simulink model "dota2_CGT"  (R2021a)
settings: Solver=VariableStepAuto  StartTime=0.0  StopTime=10.0  RelTol=1e-3
libraries: pid_lib x5, simulink x1
settings Model: Creator=srika  LastModifiedBy=srika
settings HardwareCC: TargetBitPerPointer=64  TargetBitPerSizeT=64  TargetBitPerPtrDiffT=64  TargetLongLongMode=on  TargetIntDivRoundTo=Zero  TargetEndianess=LittleEndian  TargetWordSize=64  TargetHWDeviceType=MATLAB Host  ProdEqTarget=off
settings SFSimCC: SimParseCustomCode=off
settings RTWCC: Description=Rapid Simulation Target  SystemTargetFile=rsim.tlc  TemplateMakefile=rsim_default_tmf
settings RSimTargetCC: TargetLangStandard=C99 (ISO)

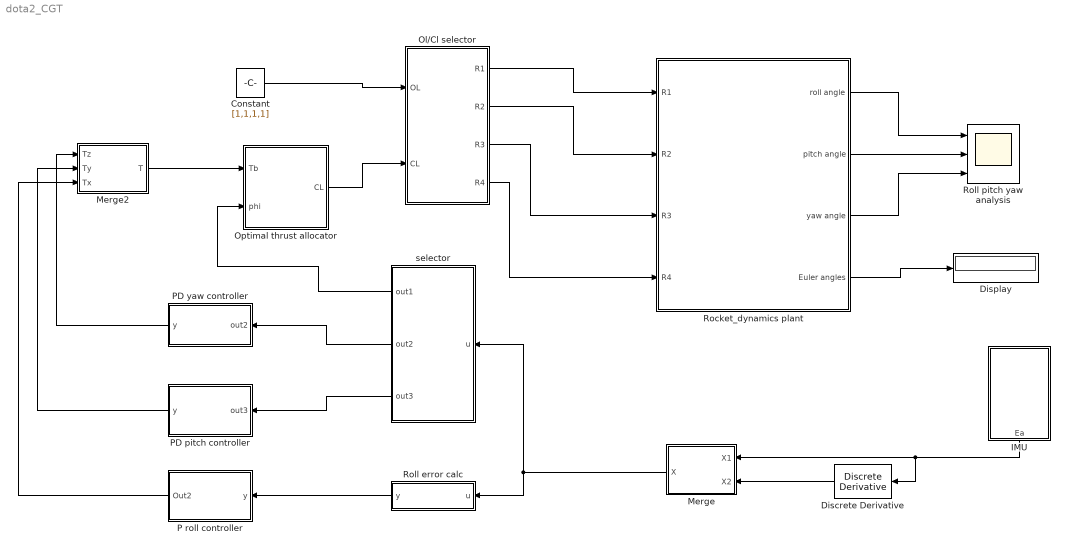
== system dota2_CGT ==
  " P roll controller" : Subsystem
  Constant : Constant  Value=[1,1,1,1]  VectorParams1D=off
  Discrete Derivative : simulink/Discrete/Discrete Derivative  gainval=1.0  ICPrevScaledInput=0.0  OutMin=[]  OutMax=[]  OutDataType=fixdt(1, 16)  OutScaling=2^-10  DoSatur=off
  Display : Display
  "IMU " : MATLAB Function  TreatAsAtomicUnit=on
  Merge : MATLAB Function  TreatAsAtomicUnit=on
  Merge2 : MATLAB Function  TreatAsAtomicUnit=on
  "Ol/Cl selector " : MATLAB Function  TreatAsAtomicUnit=on
  Optimal thrust allocator : Subsystem
  PD pitch controller : Subsystem
  PD yaw controller : Subsystem
  Rocket_dynamics plant : Subsystem
  Roll error calc : MATLAB Function  TreatAsAtomicUnit=on
  Roll pitch yaw analysis : Scope  NumInputPorts=3
  "selector " : MATLAB Function  TreatAsAtomicUnit=on
  wires:
  "IMU "/1(Ea) -> Merge/1(X1), Discrete Derivative/1
  Roll error calc/1(y) -> " P roll controller"/1(y)
  "selector "/1(out1) -> Optimal thrust allocator/2(phi)
  "selector "/2(out2) -> PD yaw controller/1(out2)
  "selector "/3(out3) -> PD pitch controller/1(out3)
  PD yaw controller/1(y) -> Merge2/1(Tz)
  PD pitch controller/1(y) -> Merge2/2(Ty)
  " P roll controller"/1(Out2) -> Merge2/3(Tx)
  Optimal thrust allocator/1(CL) -> "Ol/Cl selector "/2(CL)
  Constant/1 -> "Ol/Cl selector "/1(OL)
  "Ol/Cl selector "/1(R1) -> Rocket_dynamics plant/1(R1)
  "Ol/Cl selector "/2(R2) -> Rocket_dynamics plant/2(R2)
  "Ol/Cl selector "/3(R3) -> Rocket_dynamics plant/3(R3)
  "Ol/Cl selector "/4(R4) -> Rocket_dynamics plant/4(R4)
  Rocket_dynamics plant/1(roll angle) -> Roll pitch yaw analysis/1
  Rocket_dynamics plant/2(pitch angle) -> Roll pitch yaw analysis/2
  Rocket_dynamics plant/3(yaw angle) -> Roll pitch yaw analysis/3
  Merge2/1(T) -> Optimal thrust allocator/1(Tb)
  Discrete Derivative/1 -> Merge/2(X2)
  Merge/1(X) -> "selector "/1(u), Roll error calc/1(u)
  Rocket_dynamics plant/4(Euler angles) -> Display/1

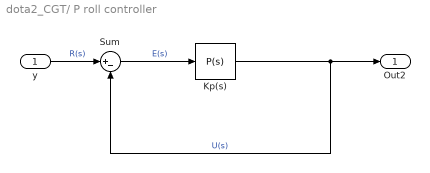
== system dota2_CGT/ P roll controller ==
  y : Inport
  Kp(s) : pid_lib/PID Controller  Controller=P  Form=Parallel  TimeDomain=Continuous-time  UseExternalTs=off  SampleTime=-1  IntegratorMethod=Forward Euler  FilterMethod=Forward Euler  ControllerParametersSource=internal  P=0.002063  I=1  D=5  UseFilter=on  N=100  TunerSelectOption=Transfer Function Based (PID Tuner App)  InitialConditionSource=internal  InitialConditionForIntegrator=0  InitialConditionForFilter=0  DifferentiatorICPrevScaledInput=0  ExternalReset=none  TrackingMode=off  Kt=1  LimitOutput=off  SatLimitsSource=internal  UpperSaturationLimit=inf  LowerSaturationLimit=-inf  LinearizeAsGain=on  AntiWindupMode=none  Kb=1  POutMin=[]  POutMax=[]  IOutMin=[]  IOutMax=[]  DOutMin=[]  DOutMax=[]  NOutMin=[]  NOutMax=[]  SumOutMin=[]  SumOutMax=[]  SaturationOutMin=[]  SaturationOutMax=[]  PParamMin=[]  PParamMax=[]  IParamMin=[]  IParamMax=[]  DParamMin=[]  DParamMax=[]  NParamMin=[]  NParamMax=[]  KbParamMin=[]  KbParamMax=[]  KtParamMin=[]  KtParamMax=[]  KbOutMin=[]  KbOutMax=[]  KtOutMin=[]  KtOutMax=[]  IntegratorOutMin=[]  IntegratorOutMax=[]  FilterOutMin=[]  FilterOutMax=[]  SumI1OutMin=[]  SumI1OutMax=[]  SumI2OutMin=[]  SumI2OutMax=[]  SumI3OutMin=[]  SumI3OutMax=[]  SumI4OutMin=[]  SumI4OutMax=[]  SumDOutMin=[]  SumDOutMax=[]  DifferentiatorOutMin=[]  DifferentiatorOutMax=[]  FilterDiffOutCoefMin=[]  FilterDiffOutCoefMax=[]  ReciprocalOutMin=[]  ReciprocalOutMax=[]  SumDenOutMin=[]  SumDenOutMax=[]  SumNumOutMin=[]  SumNumOutMax=[]  DivideOutMin=[]  DivideOutMax=[]  UdiffTsProdOutMin=[]  UdiffTsProdOutMax=[]  NTsProdOutMin=[]  NTsProdOutMax=[]  UintegralTsProdOutMin=[]  UintegralTsProdOutMax=[]  UngainTsProdOutMin=[]  UngainTsProdOutMax=[]  IntegratorContinuousStateAttributes=''  IntegratorStateMustResolveToSignalObject=off  IntegratorRTWStateStorageClass=Auto  FilterContinuousStateAttributes=''  FilterStateMustResolveToSignalObject=off  FilterRTWStateStorageClass=Auto  ParallelPVariant=InternalParameters  IdealPVariant=Disabled  IVariant=Disabled  DVariant=Disabled  IntegratorVariant=Disabled  SatVariant=Disabled  AWVariant=Disabled  PCopyVariant=Disabled  TRVariant=Disabled  FdbkBlocksVariant=Forward  IdealPFdbkVariant=Disabled  SatFdbkVariant=Disabled  DerivativeFilterVariant=Disabled  NVariant=Disabled  NCopyVariant=Disabled_SignalSpec  FilterICVariant=Disabled  IntegratorICVariant=Disabled  ExternalResetVariant=Disabled  TRSumVariant=Passthrough  SumFdbkVariant=Disabled  SumVariant=Passthrough_P  TsampFilterVariant=InternalTs  TsampNgainVariant=Passthrough  TsampIntegralVariant=Disabled_SignalSpec  ExternalSaturationOutDataTypeStr=Inherit: Same as second input
  Sum : Sum  Inputs=|+-
  Out2 : Outport
  wires:
  Sum/1 -> Kp(s)/1  "E(s)"
  Kp(s)/1 -> Sum/2, Out2/1  "U(s)"
  y/1 -> Sum/1  "R(s)"

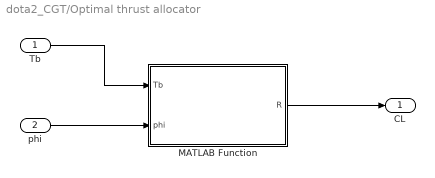
== system dota2_CGT/Optimal thrust allocator ==
  Tb : Inport
  phi : Inport  Port=2
  MATLAB Function : MATLAB Function  TreatAsAtomicUnit=on
  CL : Outport
  wires:
  Tb/1 -> MATLAB Function/1(Tb)
  phi/1 -> MATLAB Function/2(phi)
  MATLAB Function/1(R) -> CL/1

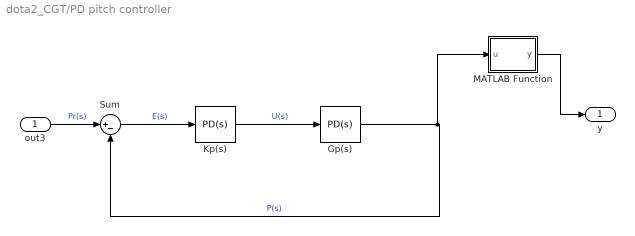
== system dota2_CGT/PD pitch controller ==
  out3 : Inport
  Gp(s) : pid_lib/PID Controller  Controller=PD  Form=Parallel  TimeDomain=Continuous-time  UseExternalTs=off  SampleTime=-1  IntegratorMethod=Forward Euler  FilterMethod=Forward Euler  ControllerParametersSource=internal  P=3  I=1  D=15  UseFilter=on  N=100  TunerSelectOption=Transfer Function Based (PID Tuner App)  InitialConditionSource=internal  InitialConditionForIntegrator=0  InitialConditionForFilter=0  DifferentiatorICPrevScaledInput=0  ExternalReset=none  TrackingMode=off  Kt=1  LimitOutput=off  SatLimitsSource=internal  UpperSaturationLimit=inf  LowerSaturationLimit=-inf  LinearizeAsGain=on  AntiWindupMode=none  Kb=1  POutMin=[]  POutMax=[]  IOutMin=[]  IOutMax=[]  DOutMin=[]  DOutMax=[]  NOutMin=[]  NOutMax=[]  SumOutMin=[]  SumOutMax=[]  SaturationOutMin=[]  SaturationOutMax=[]  PParamMin=[]  PParamMax=[]  IParamMin=[]  IParamMax=[]  DParamMin=[]  DParamMax=[]  NParamMin=[]  NParamMax=[]  KbParamMin=[]  KbParamMax=[]  KtParamMin=[]  KtParamMax=[]  KbOutMin=[]  KbOutMax=[]  KtOutMin=[]  KtOutMax=[]  IntegratorOutMin=[]  IntegratorOutMax=[]  FilterOutMin=[]  FilterOutMax=[]  SumI1OutMin=[]  SumI1OutMax=[]  SumI2OutMin=[]  SumI2OutMax=[]  SumI3OutMin=[]  SumI3OutMax=[]  SumI4OutMin=[]  SumI4OutMax=[]  SumDOutMin=[]  SumDOutMax=[]  DifferentiatorOutMin=[]  DifferentiatorOutMax=[]  FilterDiffOutCoefMin=[]  FilterDiffOutCoefMax=[]  ReciprocalOutMin=[]  ReciprocalOutMax=[]  SumDenOutMin=[]  SumDenOutMax=[]  SumNumOutMin=[]  SumNumOutMax=[]  DivideOutMin=[]  DivideOutMax=[]  UdiffTsProdOutMin=[]  UdiffTsProdOutMax=[]  NTsProdOutMin=[]  NTsProdOutMax=[]  UintegralTsProdOutMin=[]  UintegralTsProdOutMax=[]  UngainTsProdOutMin=[]  UngainTsProdOutMax=[]  IntegratorContinuousStateAttributes=''  IntegratorStateMustResolveToSignalObject=off  IntegratorRTWStateStorageClass=Auto  FilterContinuousStateAttributes=''  FilterStateMustResolveToSignalObject=off  FilterRTWStateStorageClass=Auto  ParallelPVariant=InternalParameters  IdealPVariant=Disabled  IVariant=Disabled  DVariant=InternalParameters  IntegratorVariant=Disabled  SatVariant=Disabled  AWVariant=Disabled  PCopyVariant=Disabled  TRVariant=Disabled  FdbkBlocksVariant=Forward  IdealPFdbkVariant=Disabled  SatFdbkVariant=Disabled  DerivativeFilterVariant=ContFilter  NVariant=InternalParameters  NCopyVariant=Disabled  FilterICVariant=InternalICsFilter  IntegratorICVariant=Disabled  ExternalResetVariant=Disabled  TRSumVariant=Passthrough  SumFdbkVariant=Disabled  SumVariant=Sum_PD  TsampFilterVariant=InternalTs  TsampNgainVariant=Passthrough  TsampIntegralVariant=Disabled_SignalSpec  ExternalSaturationOutDataTypeStr=Inherit: Same as second input
  Kp(s) : pid_lib/PID Controller  Controller=PD  Form=Parallel  TimeDomain=Continuous-time  UseExternalTs=off  SampleTime=-1  IntegratorMethod=Forward Euler  FilterMethod=Forward Euler  ControllerParametersSource=internal  P=3  I=1  D=5  UseFilter=on  N=100  TunerSelectOption=Transfer Function Based (PID Tuner App)  InitialConditionSource=internal  InitialConditionForIntegrator=0  InitialConditionForFilter=0  DifferentiatorICPrevScaledInput=0  ExternalReset=none  TrackingMode=off  Kt=1  LimitOutput=off  SatLimitsSource=internal  UpperSaturationLimit=inf  LowerSaturationLimit=-inf  LinearizeAsGain=on  AntiWindupMode=none  Kb=1  POutMin=[]  POutMax=[]  IOutMin=[]  IOutMax=[]  DOutMin=[]  DOutMax=[]  NOutMin=[]  NOutMax=[]  SumOutMin=[]  SumOutMax=[]  SaturationOutMin=[]  SaturationOutMax=[]  PParamMin=[]  PParamMax=[]  IParamMin=[]  IParamMax=[]  DParamMin=[]  DParamMax=[]  NParamMin=[]  NParamMax=[]  KbParamMin=[]  KbParamMax=[]  KtParamMin=[]  KtParamMax=[]  KbOutMin=[]  KbOutMax=[]  KtOutMin=[]  KtOutMax=[]  IntegratorOutMin=[]  IntegratorOutMax=[]  FilterOutMin=[]  FilterOutMax=[]  SumI1OutMin=[]  SumI1OutMax=[]  SumI2OutMin=[]  SumI2OutMax=[]  SumI3OutMin=[]  SumI3OutMax=[]  SumI4OutMin=[]  SumI4OutMax=[]  SumDOutMin=[]  SumDOutMax=[]  DifferentiatorOutMin=[]  DifferentiatorOutMax=[]  FilterDiffOutCoefMin=[]  FilterDiffOutCoefMax=[]  ReciprocalOutMin=[]  ReciprocalOutMax=[]  SumDenOutMin=[]  SumDenOutMax=[]  SumNumOutMin=[]  SumNumOutMax=[]  DivideOutMin=[]  DivideOutMax=[]  UdiffTsProdOutMin=[]  UdiffTsProdOutMax=[]  NTsProdOutMin=[]  NTsProdOutMax=[]  UintegralTsProdOutMin=[]  UintegralTsProdOutMax=[]  UngainTsProdOutMin=[]  UngainTsProdOutMax=[]  IntegratorContinuousStateAttributes=''  IntegratorStateMustResolveToSignalObject=off  IntegratorRTWStateStorageClass=Auto  FilterContinuousStateAttributes=''  FilterStateMustResolveToSignalObject=off  FilterRTWStateStorageClass=Auto  ParallelPVariant=InternalParameters  IdealPVariant=Disabled  IVariant=Disabled  DVariant=InternalParameters  IntegratorVariant=Disabled  SatVariant=Disabled  AWVariant=Disabled  PCopyVariant=Disabled  TRVariant=Disabled  FdbkBlocksVariant=Forward  IdealPFdbkVariant=Disabled  SatFdbkVariant=Disabled  DerivativeFilterVariant=ContFilter  NVariant=InternalParameters  NCopyVariant=Disabled  FilterICVariant=InternalICsFilter  IntegratorICVariant=Disabled  ExternalResetVariant=Disabled  TRSumVariant=Passthrough  SumFdbkVariant=Disabled  SumVariant=Sum_PD  TsampFilterVariant=InternalTs  TsampNgainVariant=Passthrough  TsampIntegralVariant=Disabled_SignalSpec  ExternalSaturationOutDataTypeStr=Inherit: Same as second input
  MATLAB Function : MATLAB Function  TreatAsAtomicUnit=on
  Sum : Sum  Inputs=|+-
  y : Outport
  wires:
  Gp(s)/1 -> MATLAB Function/1(u), Sum/2  "P(s)"
  Sum/1 -> Kp(s)/1  "E(s)"
  Kp(s)/1 -> Gp(s)/1  "U(s)"
  out3/1 -> Sum/1  "Pr(s)"
  MATLAB Function/1(y) -> y/1

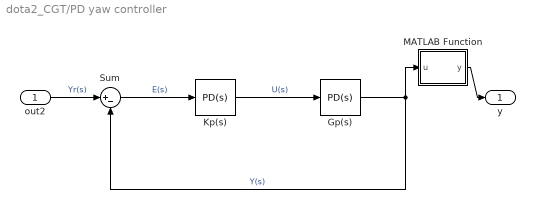
== system dota2_CGT/PD yaw controller ==
  out2 : Inport
  Gp(s) : pid_lib/PID Controller  Controller=PD  Form=Parallel  TimeDomain=Continuous-time  UseExternalTs=off  SampleTime=-1  IntegratorMethod=Forward Euler  FilterMethod=Forward Euler  ControllerParametersSource=internal  P=3  I=1  D=15  UseFilter=on  N=100  TunerSelectOption=Transfer Function Based (PID Tuner App)  InitialConditionSource=internal  InitialConditionForIntegrator=0  InitialConditionForFilter=0  DifferentiatorICPrevScaledInput=0  ExternalReset=none  TrackingMode=off  Kt=1  LimitOutput=off  SatLimitsSource=internal  UpperSaturationLimit=inf  LowerSaturationLimit=-inf  LinearizeAsGain=on  AntiWindupMode=none  Kb=1  POutMin=[]  POutMax=[]  IOutMin=[]  IOutMax=[]  DOutMin=[]  DOutMax=[]  NOutMin=[]  NOutMax=[]  SumOutMin=[]  SumOutMax=[]  SaturationOutMin=[]  SaturationOutMax=[]  PParamMin=[]  PParamMax=[]  IParamMin=[]  IParamMax=[]  DParamMin=[]  DParamMax=[]  NParamMin=[]  NParamMax=[]  KbParamMin=[]  KbParamMax=[]  KtParamMin=[]  KtParamMax=[]  KbOutMin=[]  KbOutMax=[]  KtOutMin=[]  KtOutMax=[]  IntegratorOutMin=[]  IntegratorOutMax=[]  FilterOutMin=[]  FilterOutMax=[]  SumI1OutMin=[]  SumI1OutMax=[]  SumI2OutMin=[]  SumI2OutMax=[]  SumI3OutMin=[]  SumI3OutMax=[]  SumI4OutMin=[]  SumI4OutMax=[]  SumDOutMin=[]  SumDOutMax=[]  DifferentiatorOutMin=[]  DifferentiatorOutMax=[]  FilterDiffOutCoefMin=[]  FilterDiffOutCoefMax=[]  ReciprocalOutMin=[]  ReciprocalOutMax=[]  SumDenOutMin=[]  SumDenOutMax=[]  SumNumOutMin=[]  SumNumOutMax=[]  DivideOutMin=[]  DivideOutMax=[]  UdiffTsProdOutMin=[]  UdiffTsProdOutMax=[]  NTsProdOutMin=[]  NTsProdOutMax=[]  UintegralTsProdOutMin=[]  UintegralTsProdOutMax=[]  UngainTsProdOutMin=[]  UngainTsProdOutMax=[]  IntegratorContinuousStateAttributes=''  IntegratorStateMustResolveToSignalObject=off  IntegratorRTWStateStorageClass=Auto  FilterContinuousStateAttributes=''  FilterStateMustResolveToSignalObject=off  FilterRTWStateStorageClass=Auto  ParallelPVariant=InternalParameters  IdealPVariant=Disabled  IVariant=Disabled  DVariant=InternalParameters  IntegratorVariant=Disabled  SatVariant=Disabled  AWVariant=Disabled  PCopyVariant=Disabled  TRVariant=Disabled  FdbkBlocksVariant=Forward  IdealPFdbkVariant=Disabled  SatFdbkVariant=Disabled  DerivativeFilterVariant=ContFilter  NVariant=InternalParameters  NCopyVariant=Disabled  FilterICVariant=InternalICsFilter  IntegratorICVariant=Disabled  ExternalResetVariant=Disabled  TRSumVariant=Passthrough  SumFdbkVariant=Disabled  SumVariant=Sum_PD  TsampFilterVariant=InternalTs  TsampNgainVariant=Passthrough  TsampIntegralVariant=Disabled_SignalSpec  ExternalSaturationOutDataTypeStr=Inherit: Same as second input
  Kp(s) : pid_lib/PID Controller  Controller=PD  Form=Parallel  TimeDomain=Continuous-time  UseExternalTs=off  SampleTime=-1  IntegratorMethod=Forward Euler  FilterMethod=Forward Euler  ControllerParametersSource=internal  P=3  I=1  D=5  UseFilter=on  N=100  TunerSelectOption=Transfer Function Based (PID Tuner App)  InitialConditionSource=internal  InitialConditionForIntegrator=0  InitialConditionForFilter=0  DifferentiatorICPrevScaledInput=0  ExternalReset=none  TrackingMode=off  Kt=1  LimitOutput=off  SatLimitsSource=internal  UpperSaturationLimit=inf  LowerSaturationLimit=-inf  LinearizeAsGain=on  AntiWindupMode=none  Kb=1  POutMin=[]  POutMax=[]  IOutMin=[]  IOutMax=[]  DOutMin=[]  DOutMax=[]  NOutMin=[]  NOutMax=[]  SumOutMin=[]  SumOutMax=[]  SaturationOutMin=[]  SaturationOutMax=[]  PParamMin=[]  PParamMax=[]  IParamMin=[]  IParamMax=[]  DParamMin=[]  DParamMax=[]  NParamMin=[]  NParamMax=[]  KbParamMin=[]  KbParamMax=[]  KtParamMin=[]  KtParamMax=[]  KbOutMin=[]  KbOutMax=[]  KtOutMin=[]  KtOutMax=[]  IntegratorOutMin=[]  IntegratorOutMax=[]  FilterOutMin=[]  FilterOutMax=[]  SumI1OutMin=[]  SumI1OutMax=[]  SumI2OutMin=[]  SumI2OutMax=[]  SumI3OutMin=[]  SumI3OutMax=[]  SumI4OutMin=[]  SumI4OutMax=[]  SumDOutMin=[]  SumDOutMax=[]  DifferentiatorOutMin=[]  DifferentiatorOutMax=[]  FilterDiffOutCoefMin=[]  FilterDiffOutCoefMax=[]  ReciprocalOutMin=[]  ReciprocalOutMax=[]  SumDenOutMin=[]  SumDenOutMax=[]  SumNumOutMin=[]  SumNumOutMax=[]  DivideOutMin=[]  DivideOutMax=[]  UdiffTsProdOutMin=[]  UdiffTsProdOutMax=[]  NTsProdOutMin=[]  NTsProdOutMax=[]  UintegralTsProdOutMin=[]  UintegralTsProdOutMax=[]  UngainTsProdOutMin=[]  UngainTsProdOutMax=[]  IntegratorContinuousStateAttributes=''  IntegratorStateMustResolveToSignalObject=off  IntegratorRTWStateStorageClass=Auto  FilterContinuousStateAttributes=''  FilterStateMustResolveToSignalObject=off  FilterRTWStateStorageClass=Auto  ParallelPVariant=InternalParameters  IdealPVariant=Disabled  IVariant=Disabled  DVariant=InternalParameters  IntegratorVariant=Disabled  SatVariant=Disabled  AWVariant=Disabled  PCopyVariant=Disabled  TRVariant=Disabled  FdbkBlocksVariant=Forward  IdealPFdbkVariant=Disabled  SatFdbkVariant=Disabled  DerivativeFilterVariant=ContFilter  NVariant=InternalParameters  NCopyVariant=Disabled  FilterICVariant=InternalICsFilter  IntegratorICVariant=Disabled  ExternalResetVariant=Disabled  TRSumVariant=Passthrough  SumFdbkVariant=Disabled  SumVariant=Sum_PD  TsampFilterVariant=InternalTs  TsampNgainVariant=Passthrough  TsampIntegralVariant=Disabled_SignalSpec  ExternalSaturationOutDataTypeStr=Inherit: Same as second input
  MATLAB Function : MATLAB Function  TreatAsAtomicUnit=on
  Sum : Sum  Inputs=|+-
  y : Outport
  wires:
  Kp(s)/1 -> Gp(s)/1  "U(s)"
  Sum/1 -> Kp(s)/1  "E(s)"
  out2/1 -> Sum/1  "Yr(s)"
  Gp(s)/1 -> MATLAB Function/1(u), Sum/2  "Y(s)"
  MATLAB Function/1(y) -> y/1

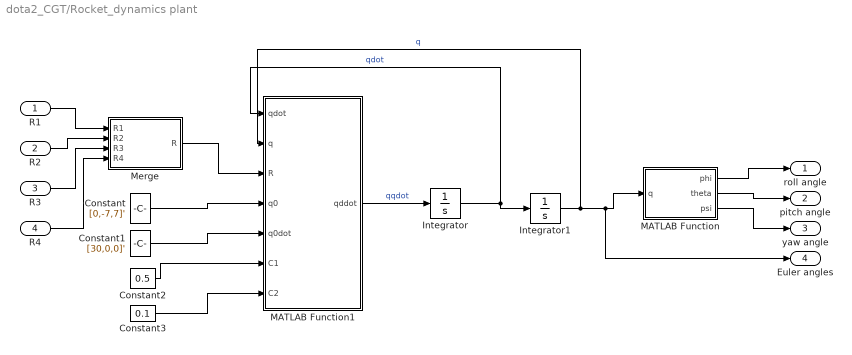
== system dota2_CGT/Rocket_dynamics plant ==
  R1 : Inport
  R2 : Inport  Port=2
  R3 : Inport  Port=3
  R4 : Inport  Port=4
  Constant : Constant  Value=[0,-7,7]'
  Constant1 : Constant  Value=[30,0,0]'
  Constant2 : Constant  Value=0.5
  Constant3 : Constant  Value=0.1
  Integrator : Integrator
  Integrator1 : Integrator
  MATLAB Function : MATLAB Function  TreatAsAtomicUnit=on
  MATLAB Function1 : MATLAB Function  TreatAsAtomicUnit=on
  Merge : MATLAB Function  TreatAsAtomicUnit=on
  roll angle : Outport
  pitch angle : Outport  Port=2
  yaw angle : Outport  Port=3
  Euler angles : Outport  Port=4
  wires:
  Constant3/1 -> MATLAB Function1/7(C2)
  Constant1/1 -> MATLAB Function1/5(q0dot)
  Merge/1(R) -> MATLAB Function1/3(R)
  Integrator/1 -> Integrator1/1, MATLAB Function1/1(qdot)  "qdot"
  R2/1 -> Merge/2(R2)
  MATLAB Function/2(theta) -> pitch angle/1
  Integrator1/1 -> MATLAB Function1/2(q), Euler angles/1, MATLAB Function/1(q)  "q"
  MATLAB Function/1(phi) -> roll angle/1
  MATLAB Function/3(psi) -> yaw angle/1
  R1/1 -> Merge/1(R1)
  R3/1 -> Merge/3(R3)
  MATLAB Function1/1(qddot) -> Integrator/1  "qqdot"
  Constant2/1 -> MATLAB Function1/6(C1)
  Constant/1 -> MATLAB Function1/4(q0)
  R4/1 -> Merge/4(R4)

== matlab function dota2_CGT/PD yaw controller/MATLAB Function ==
  data: u input; y output
function y = fcn(u)

y = u(1);

== matlab function dota2_CGT/PD pitch controller/MATLAB Function ==
  data: u input; y output
function y = fcn(u)

y = u(1);

== matlab function dota2_CGT/IMU  ==
  data: Ea output
function Ea= imu()
    %data_log=zeros(1,20);
    %data_log = readtable("imu_data.csv");
    %Ea=data_log(1,3:5);
    Ea=[3.14/6,3.14/4,3.14/8];

== matlab function dota2_CGT/Optimal thrust allocator/MATLAB Function ==
  data: Tb input; R output; phi input
function R = fcn(Tb,phi)
R=[0,0,0,0];
%input parameters
minratio=0;
pivotrow=[0,0,0,0,0,0,0,0];
pivotcol=[0,0,0,0]
h=0.4;
Noofvariables=4;
f=0.01;
C=[1,1,1,1];
info=[-sin(phi),-cos(phi),sin(phi),cos(phi);-cos(phi),sin(phi),cos(phi),-sin(phi);-f,f,-f,f];
s=eye(3);
b=[Tb(3)/h,Tb(2)/h,Tb(1)]';
tableS=zeros(4,8);


%computation
A=[info,s,b];
Cost=zeros(1,size(A,2));
Cost(1:Noofvariables)=C;
BV=5:1:7;
zjcj=Cost(BV)*A-Cost;
BFS=zeros(1,size(A,2));
zcj=[zjcj;A];
tableS=array2table(zcj,'VariableNames',{'x_1','x_2','x_3','x_4','s_1','s_2','s_3','solu'});
%tableS=array2table(zcj);
%tableS.Properties.VariableNames(1:size(zcj,2))={'x_1','x_2','x_3','x_4','s_1','s_2','s_3','solu'};
zc=zjcj(1:size(zjcj,2)-1);
run=true;
while run
    if any(zjcj<0)
        [minvalue,pivotcol]=min(zc);
        sol=A(:,end);
        column=A(:,pivotcol);
        ratio=zeros(1,3);
        for i=1:size(column,1)
            if column(i)>0
                ratio(i)=sol(i)./column(i);
            else
                ratio(i)=inf;
            end
        end
        %finding the pivot row
        [minratio,pivotrow]=min(ratio);
        BV(pivotrow)=pivotcol;
        pivotkey=A(pivotrow,pivotcol);
        %A(pivotrow,:) = A(pivotrow,:)/pivotkey;
        for i=1:size(A,2)
            A(pivotrow,i)=A(pivotrow,i)/pivotkey;
        end
        for i=1:size(A,1)
            if i~=pivotrow
                A(i,:)=A(i,:)-A(i,pivotcol).*A(pivotrow,:);
            end
                zjcj=zjcj-zjcj(pivotcol).*A(pivotrow,:);
        end 
        
        zcj=[zjcj;A];
        tableS=array2table(zcj,'VariableNames',{'x_1','x_2','x_3','x_4','s_1','s_2','s_3','solu'});
        %tableS.Properties.VariableNames(1:size(zcj,2))={'x_1','x_2','x_3','x_4','s_1','s_2','s_3','solu'};
        
        BFS(BV)=A(:,end);
        BFS(end)=sum(BFS.*Cost);
        CurrentBFS=array2table(BFS,'VariableNames',{'x_1','x_2','x_3','x_4','s_1','s_2','s_3','solu'});
        %CurrentBFS=array2table(BFS);
        %CurrentBFS.Properties.VariableNames(1:size(CurrentBFS,2))={'x_1','x_2','x_3','x_4','s_1','s_2','s_3','solu'};
    else
        run=false;
        R=BFS(1:4);
  
    end
end

== matlab function dota2_CGT/Ol//Cl selector  ==
  data: OL input; R1 output; R2 output; R3 output; CL input; R4 output
function [R1,R2,R3,R4] = fcn(OL,CL)
if OL(1)>CL(1)
    R1=CL(1);
else
    R1=OL(1);
end

if OL(2)>CL(2)
    R2=CL(2);
else
    R2=OL(2);
end
if OL(3)>CL(3)
    R3=CL(3);
else
    R3=OL(3);
end
if OL(4)>CL(4)
    R4=CL(4);
else
    R4=OL(4);
end

== matlab function dota2_CGT/Roll error calc ==
  data: u input; y output
function y = fcn(u)

y = u(4)-u(6)*sin(u(2));

== matlab function dota2_CGT/selector  ==
  data: u input; out1 output; out2 output; out3 output
function [out1,out2,out3] = fcn(u)

out1 = [u(1)];
out2 = [u(3),u(6)];
out3 = [u(2),u(5)];

== matlab function dota2_CGT/Rocket_dynamics plant/MATLAB Function1 ==
  data: qdot input; qddot output; q input; R input; q0 input; q0dot input; C1 input; C2 input
function qddot  = fcn(qdot,q,R,q0,q0dot,C1,C2)
% this function will calculate the 2nd order derivative of q(qddot) using
%   the equation M(q)*qddot + C(q,qdot) + G(q)=F(q)
% Each of these terms has to be calculated first before proceeding to the
%   calcutation of qddot
%--------------------------------------------
% 1.setup
    qddot=[0,0,0]';
    J=[1,0,0;0,1,0;0,0,1];
    h=0.4;
    f=0.01;
    A1=[0,0,0;0,-C1,0;0,0,-C1];
    A2=[0,0,0;0,-C2,0;0,0,-C2];
    W=[1,0,-sin(q(2));0,-cos(q(1)),sin(q(1))*cos(q(2));0,-sin(q(1)),cos(q(1))*cos(q(2))];
    B=[-f,f,-f,f;-h,0,h,0;0,-h,0,h];
    

%--------------------------------------------
% 2.calculation of F(q) using formula F(q)=T(q)+A(q)
    A=A1*(q-q0) +A2*(qdot-q0dot);
    T=W*B*R;
    F=T+A;
%--------------------------------------------
% 3. Calculation of M(q) 
    M=transpose(W)*J*W;
%--------------------------------------------
% 4. Calculation of C(q,qdot)
    i=1;
    j=1;
    k=1;
    for i=1:3
        for j=1:3
            for k=1:3
                C(i,j)=0.5*((diff(M(i,j))/diff(q(k)))+(diff(M(i,j))/diff(q(k)))-(diff(M(i,j))/diff(q(k))))
    
%--------------------------------------------
% 5. final calculation 
    syms t;
    ode=M*diff(diff(q(1),t))+C*diff(q(1),t)==F;
    qddot(1)=dsolve(ode);
    ode=M*diff(diff(q(2),t))+C*diff(q(2),t)==F;
    qddot(2)=dsolve(ode);
    ode=M*diff(diff(q(3),t))+C*diff(q(3),t)==F;
    qddot(3)=dsolve(ode);

== matlab function dota2_CGT/Rocket_dynamics plant/MATLAB Function ==
  data: phi output; theta output; q input; psi output
function [phi,theta,psi] = fcn(q)
phi=q(1);
theta=q(2);
psi=q(3);

== matlab function dota2_CGT/Rocket_dynamics plant/Merge ==
  data: R1 input; R output; R2 input; R3 input; R4 input
function R = fcn(R1,R2,R3,R4)
R=[0,0,0,0]';
R(1)=R1;
R(2)=R2;
R(3)=R3;
R(4)=R4;

== matlab function dota2_CGT/Merge2 ==
  data: Tz input; Ty input; Tx input; T output
function T = fcn(Tz,Ty,Tx)
T=[Tx,Ty,Tz];

== matlab function dota2_CGT/Merge ==
  data: X1 input; X2 input; X output
function X=fcn(X1,X2)
X=[0,0,0,0,0,0];
X(1)=X1(1);
X(2)=X1(2);
X(3)=X1(3);
X(4)=X2(1);
X(5)=X2(2);
X(6)=X2(3);
